simulink library "sm_trackV_lib_belt_contact"  (R2026a)
settings: Solver=VariableStepAuto
undefined symbols (not defined in the file): Scene, Trac
libraries: sm_lib x3
Description:
  | Copyright 2024-2026 The MathWorks, Inc.
settings Model: Creator=smiller  LastModifiedBy=smiller

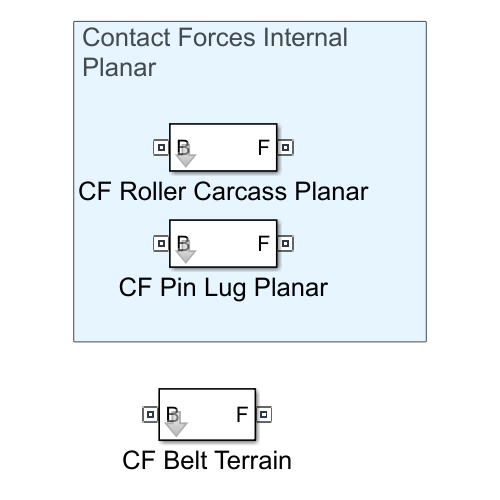
[thumbnail: Simulink's stored preview of the top-level diagram]
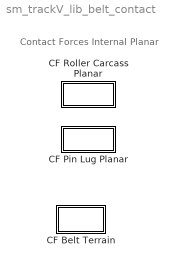
== system sm_trackV_lib_belt_contact ==
  note: Contact Forces Internal
      | Planar
  CF Belt Terrain : Subsystem  mask(Contact Force, Belt Segment to Terrain){NormalStiffness=Scene.Contact.Terrain.K, NormalDamping=Scene.Contact.Terrain.B, NormalTransitionRegionWidth=Scene.Contact.Terrain.TW, CoefficientOfDynamicFriction=Scene.Contact.Terrain.mud, CoefficientOfStaticFriction=Scene.Contact.Terrain.mus, FrictionalCriticalVelocity=Scene.Contact.Terrain.CV}
      mask prompts: NormalStiffness "Normal Stiffness (N/m)"; NormalDamping "Normal Damping (N/(m/s))"; NormalTransitionRegionWidth "Normal Transition Width (m)"; CoefficientOfDynamicFriction "Coefficient of Dynamic Friction"; CoefficientOfStaticFriction "Coefficient of Static Friction"; FrictionalCriticalVelocity "Critical Velocity (m/s)"
      mask help: Models contact force between one belt segment and the terrain.
      mask TypeOptions NormalStiffness:
      | Spatial
      | Contact Force/NormalStiffness
      mask TypeOptions NormalDamping:
      | Spatial
      | Contact Force/NormalDamping
      mask TypeOptions NormalTransitionRegionWidth:
      | Spatial
      | Contact Force/NormalTransitionRegionWidth
      mask TypeOptions CoefficientOfDynamicFriction:
      | Spatial
      | Contact Force/CoefficientOfDynamicFriction
      mask TypeOptions CoefficientOfStaticFriction:
      | Spatial
      | Contact Force/CoefficientOfStaticFriction
      mask TypeOptions FrictionalCriticalVelocity:
      | Spatial
      | Contact Force/FrictionalCriticalVelocity
  CF Pin Lug Planar : Subsystem  mask(Contact Force between Lug and Sprocket Pin (Planar)){K_SprocketLug=Trac.Contact.SprocketLug.K, B_SprocketLug=Trac.Contact.SprocketLug.B, TW_SprocketLug=Trac.Contact.SprocketLug.TW}
      mask prompts: K_SprocketLug "Normal Stiffness (N/m)"; B_SprocketLug "Normal Damping (N/(m/s))"; TW_SprocketLug "Normal Transition Width (m)"
      mask help: Models contact force between one lug and one sprocket pin. Assumes planar contact.
      mask TypeOptions K_SprocketLug:
      | Planar
      | Contact Force/NormalStiffness
      mask TypeOptions B_SprocketLug:
      | Planar
      | Contact Force/NormalDamping
      mask TypeOptions TW_SprocketLug:
      | Planar
      | Contact Force/NormalTransitionRegionWidth
  CF Roller Carcass Planar : Subsystem  mask(Contact Force between Belt and Roller (Planar)){K_Roller=1e7, B_Roller=1e5, TW_Roller=1e-3}
      mask prompts: K_Roller "Normal Stiffness (N/m)"; B_Roller "Normal Damping (N/(m/s))"; TW_Roller "Normal Transition Width (m)"
      mask help: Models contact force between one belt segment and a roller. Assumes planar contact.
      mask TypeOptions K_Roller:
      | Planar
      | Contact Force/NormalStiffness
      mask TypeOptions B_Roller:
      | Planar
      | Contact Force/NormalDamping
      mask TypeOptions TW_Roller:
      | Planar
      | Contact Force/NormalTransitionRegionWidth

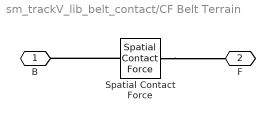
== system sm_trackV_lib_belt_contact/CF Belt Terrain ==
  Spatial Contact Force : sm_lib/Forces and Torques/Spatial Contact Force  SenseSeparationDistance=off  NormalForceType=SmoothSpringDamper  NormalStiffness=NormalStiffness  NormalStiffnessUnits=N/m  NormalDamping=NormalDamping  NormalDampingUnits=N/(m/s)  NormalTransitionRegionWidth=NormalTransitionRegionWidth  NormalTransitionRegionWidthUnits=m  FrictionType=SmoothStickSlip  CoefficientOfStaticFriction=CoefficientOfStaticFriction  CoefficientOfDynamicFriction=CoefficientOfDynamicFriction  FrictionalCriticalVelocity=FrictionalCriticalVelocity  FrictionalCriticalVelocityUnits=m/s  SenseContactSignal=off  SensePenetrationDepth=off  SenseNormalVelocity=off  SenseTangentialVelocity=off  SensingForceTorqueDirection=BaseOnFollower  SensingForceTorqueResolutionFrame=ContactFrame  SenseNormalForce=off  SenseNormalForceMagnitude=off  SenseNormalTorque=off  SenseFrictionalForce=off  SenseFrictionalForceMagnitude=off  SenseFrictionalTorque=off  SenseTotalForce=off  SenseTotalTorque=off  SenseContactBaseRotation=off  SenseContactBaseTranslation=off  SenseContactFollowerRotation=off  SenseContactFollowerTranslation=off  ZeroCrossDetectContactStartAndEnd=off
  B : PMIOPort  Side=Left
  F : PMIOPort  Port=2  Side=Right
  connections:
  Spatial Contact Force/RConn1 -- F/RConn1
  Spatial Contact Force/LConn1 -- B/RConn1

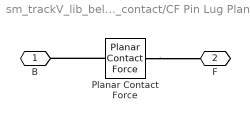
== system sm_trackV_lib_belt_contact/CF Pin Lug Planar ==
  Planar Contact Force : sm_lib/Forces and Torques/Planar Contact Force  NormalForceType=SmoothSpringDamper  NormalStiffness=K_SprocketLug  NormalStiffnessUnits=N/m  NormalDamping=B_SprocketLug  NormalDampingUnits=N/(m/s)  NormalTransitionRegionWidth=TW_SprocketLug  NormalTransitionRegionWidthUnits=m  FrictionType=None  CoefficientOfStaticFriction=0.5  CoefficientOfDynamicFriction=0.3  FrictionalCriticalVelocity=1e-3  FrictionalCriticalVelocityUnits=m/s  SenseContactSignal=off  SensePenetrationDepth=off  SenseNormalVelocity=off  SenseTangentialVelocity=off  SensingForceTorqueDirection=BaseOnFollower  SensingForceTorqueResolutionFrame=ContactFrame  SenseNormalForce=off  SenseNormalForceMagnitude=off  SenseNormalTorque=off  SenseFrictionalForce=off  SenseFrictionalForceMagnitude=off  SenseFrictionalTorque=off  SenseTotalForce=off  SenseTotalTorque=off  SenseContactBaseRotation=off  SenseContactBaseTranslation=off  SenseContactFollowerRotation=off  SenseContactFollowerTranslation=off  ZeroCrossDetectContactStartAndEnd=off
  B : PMIOPort  Side=Left
  F : PMIOPort  Port=2  Side=Right
  connections:
  Planar Contact Force/RConn1 -- F/RConn1
  Planar Contact Force/LConn1 -- B/RConn1

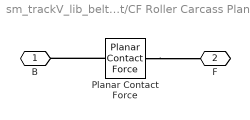
== system sm_trackV_lib_belt_contact/CF Roller Carcass Planar ==
  Planar Contact Force : sm_lib/Forces and Torques/Planar Contact Force  NormalForceType=SmoothSpringDamper  NormalStiffness=K_Roller  NormalStiffnessUnits=N/m  NormalDamping=B_Roller  NormalDampingUnits=N/(m/s)  NormalTransitionRegionWidth=TW_Roller  NormalTransitionRegionWidthUnits=m  FrictionType=None  CoefficientOfStaticFriction=0.5  CoefficientOfDynamicFriction=0.3  FrictionalCriticalVelocity=1e-3  FrictionalCriticalVelocityUnits=m/s  SenseContactSignal=off  SensePenetrationDepth=off  SenseNormalVelocity=off  SenseTangentialVelocity=off  SensingForceTorqueDirection=BaseOnFollower  SensingForceTorqueResolutionFrame=ContactFrame  SenseNormalForce=off  SenseNormalForceMagnitude=off  SenseNormalTorque=off  SenseFrictionalForce=off  SenseFrictionalForceMagnitude=off  SenseFrictionalTorque=off  SenseTotalForce=off  SenseTotalTorque=off  SenseContactBaseRotation=off  SenseContactBaseTranslation=off  SenseContactFollowerRotation=off  SenseContactFollowerTranslation=off  ZeroCrossDetectContactStartAndEnd=off
  B : PMIOPort  Side=Left
  F : PMIOPort  Port=2  Side=Right
  connections:
  Planar Contact Force/LConn1 -- B/RConn1
  Planar Contact Force/RConn1 -- F/RConn1
